simulink model "model"  (R2024a)
settings: Solver=VariableStepAuto  StartTime=0.0  StopTime=20  RelTol=1e-3
undefined symbols (not defined in the file): Kp, Td, Ti
libraries: cstblocks x1
settings Model: SimulationMode=accelerator  Creator=thoma  LastModifiedBy=thoma

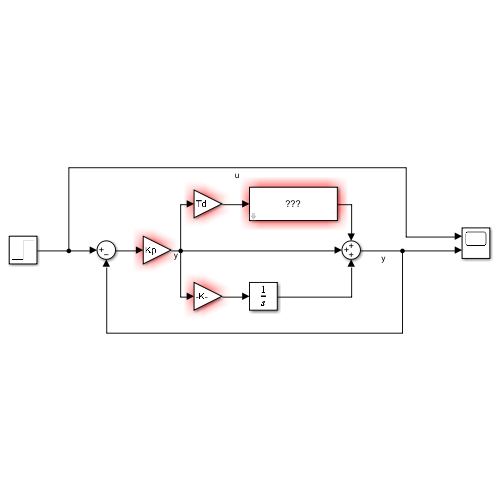
[thumbnail: Simulink's stored preview of the top-level diagram]
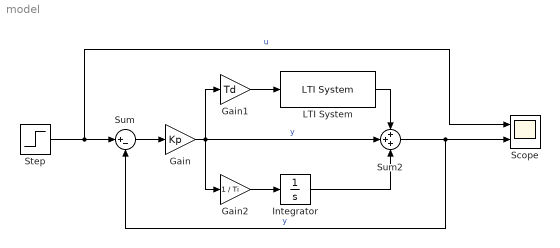
== system model ==
  Gain : Gain  Gain=Kp
  Gain1 : Gain  Gain=Td
  Gain2 : Gain  Gain=1 / Ti
  Integrator : Integrator
  LTI System : cstblocks/LTI System  sys=F  IC=[]  PadeOrder=0
  Scope : Scope  NumInputPorts=2
  Step : Step  SampleTime=0
  Sum : Sum  Inputs=|+-
  Sum2 : Sum  Inputs=+++
  wires:
  Gain/1 -> Gain2/1, Sum2/2, Gain1/1  "y"
  Step/1 -> Sum/1, Scope/1  "u"
  Sum/1 -> Gain/1
  Gain1/1 -> LTI System/1
  Gain2/1 -> Integrator/1
  Integrator/1 -> Sum2/3
  LTI System/1 -> Sum2/1
  Sum2/1 -> Sum/2, Scope/2  "y"
